simulink model "IO324_src"  (R2022b)
settings: Solver=FixedStepDiscrete  StartTime=0.0  StopTime=10.0  RelTol=1e-3
libraries: SG_library x1, hdlsllib x1
settings Model: DataTypeOverride=Off  Creator=mavolery  LastModifiedBy=mavolery
settings OptimizationCC: BlockReduction=off  ConditionallyExecuteInputs=off  DefaultParameterBehavior=Inlined  InheritOutputTypeSmallerThanSingle=on
settings DebuggingCC: AlgebraicLoopMsg=error  InheritedTsInSrcMsg=none  SingleTaskRateTransMsg=error
settings HardwareCC: ProdBitPerPointer=32  ProdBitPerSizeT=32  ProdBitPerPtrDiffT=32  ProdLargestAtomicFloat=None  ProdIntDivRoundTo=Undefined  ProdEndianess=Unspecified  ProdWordSize=32  ProdHWDeviceType=ASIC/FPGA->ASIC/FPGA  TargetBitPerPointer=64  TargetBitPerSizeT=64  TargetBitPerPtrDiffT=64  TargetLongLongMode=on  TargetIntDivRoundTo=Zero  TargetEndianess=LittleEndian  TargetWordSize=64  TargetHWDeviceType=Custom Processor->MATLAB Host Computer  ProdEqTarget=off

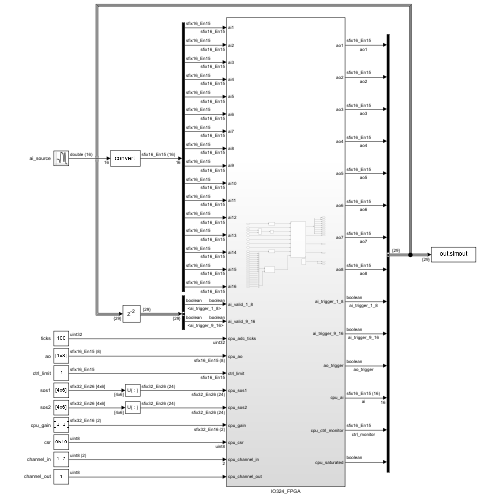
[thumbnail: Simulink's stored preview of the top-level diagram]
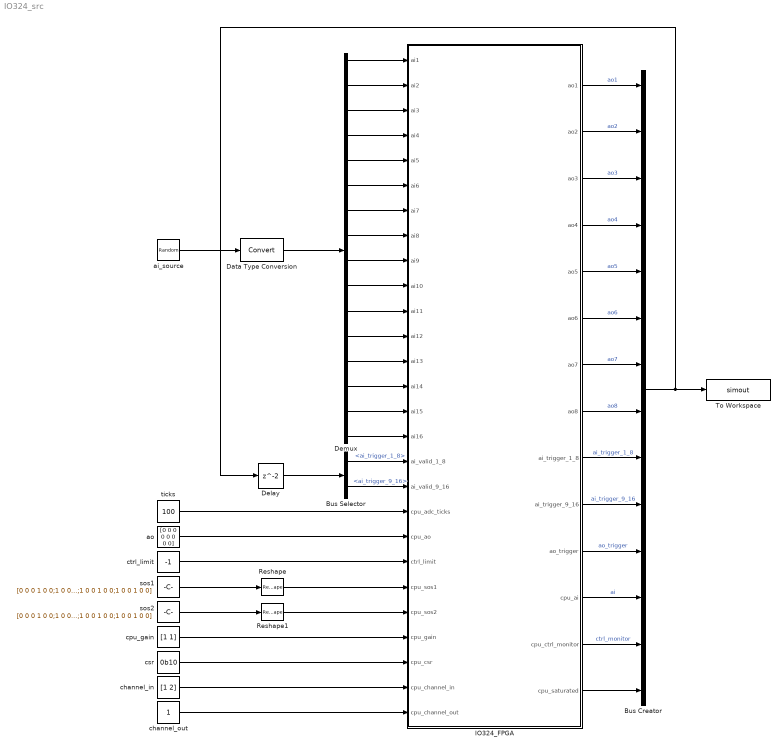
== system IO324_src ==
  Bus Creator : BusCreator  Inputs=14
  Bus Selector : BusSelector  OutputSignals=ai_trigger_1_8,ai_trigger_9_16
  Data Type Conversion : DataTypeConversion  SaturateOnIntegerOverflow=off  RndMeth=Floor
  Delay : Delay
  Demux : Demux  Outputs=16
  IO324_FPGA : Subsystem
  Reshape : Reshape
  Reshape1 : Reshape
  To Workspace : ToWorkspace  VariableName=simout  SaveFormat=Timeseries  SampleTime=-1
  ai_source : RandomNumber  Variance=1e-3  Seed=0:15
  ao : Constant  Value=[0 0 0 0 0 0 0 0]  OutDataTypeStr=Inherit: Inherit via back propagation  SampleTime=-1
  channel_in : Constant  Value=[1 2]  OutDataTypeStr=Inherit: Inherit via back propagation  SampleTime=-1
  channel_out : Constant  OutDataTypeStr=Inherit: Inherit via back propagation  SampleTime=-1
  cpu_gain : Constant  Value=[1 1]  OutDataTypeStr=Inherit: Inherit via back propagation  SampleTime=-1
  csr : Constant  Value=0b10  OutDataTypeStr=Inherit: Inherit via back propagation  SampleTime=-1
  ctrl_limit : Constant  Value=-1  OutDataTypeStr=Inherit: Inherit via back propagation  SampleTime=-1
  sos1 : Constant  Value=[0 0 0 1 0 0;1 0 0 1 0 0;1 0 0 1 0 0;1 0 0 1 0 0]  OutDataTypeStr=Inherit: Inherit via back propagation  SampleTime=-1
  sos2 : Constant  Value=[0 0 0 1 0 0;1 0 0 1 0 0;1 0 0 1 0 0;1 0 0 1 0 0]  OutDataTypeStr=Inherit: Inherit via back propagation  SampleTime=-1
  ticks : Constant  Value=100  OutDataTypeStr=Inherit: Inherit via back propagation  SampleTime=-1
  wires:
  Bus Creator/1 -> To Workspace/1, Delay/1
  IO324_FPGA/12(cpu_ai) -> Bus Creator/12  "ai"
  Reshape/1 -> IO324_FPGA/22(cpu_sos1)
  IO324_FPGA/4(ao4) -> Bus Creator/4  "ao4"
  IO324_FPGA/8(ao8) -> Bus Creator/8  "ao8"
  IO324_FPGA/1(ao1) -> Bus Creator/1  "ao1"
  ctrl_limit/1 -> IO324_FPGA/21(ctrl_limit)
  IO324_FPGA/3(ao3) -> Bus Creator/3  "ao3"
  IO324_FPGA/11(ao_trigger) -> Bus Creator/11  "ao_trigger"
  IO324_FPGA/2(ao2) -> Bus Creator/2  "ao2"
  IO324_FPGA/7(ao7) -> Bus Creator/7  "ao7"
  IO324_FPGA/10(ai_trigger_9_16) -> Bus Creator/10  "ai_trigger_9_16"
  IO324_FPGA/9(ai_trigger_1_8) -> Bus Creator/9  "ai_trigger_1_8"
  IO324_FPGA/13(cpu_ctrl_monitor) -> Bus Creator/13  "ctrl_monitor"
  ticks/1 -> IO324_FPGA/19(cpu_adc_ticks)
  IO324_FPGA/6(ao6) -> Bus Creator/6  "ao6"
  sos2/1 -> Reshape1/1
  csr/1 -> IO324_FPGA/25(cpu_csr)
  cpu_gain/1 -> IO324_FPGA/24(cpu_gain)
  sos1/1 -> Reshape/1
  Reshape1/1 -> IO324_FPGA/23(cpu_sos2)
  IO324_FPGA/5(ao5) -> Bus Creator/5  "ao5"
  ai_source/1 -> Data Type Conversion/1
  ao/1 -> IO324_FPGA/20(cpu_ao)
  Demux/1 -> IO324_FPGA/1(ai1)
  Demux/2 -> IO324_FPGA/2(ai2)
  Demux/3 -> IO324_FPGA/3(ai3)
  Demux/4 -> IO324_FPGA/4(ai4)
  Demux/5 -> IO324_FPGA/5(ai5)
  Demux/6 -> IO324_FPGA/6(ai6)
  Demux/7 -> IO324_FPGA/7(ai7)
  Demux/8 -> IO324_FPGA/8(ai8)
  Demux/9 -> IO324_FPGA/9(ai9)
  Demux/10 -> IO324_FPGA/10(ai10)
  Demux/11 -> IO324_FPGA/11(ai11)
  Demux/12 -> IO324_FPGA/12(ai12)
  Demux/13 -> IO324_FPGA/13(ai13)
  Demux/14 -> IO324_FPGA/14(ai14)
  Demux/15 -> IO324_FPGA/15(ai15)
  Demux/16 -> IO324_FPGA/16(ai16)
  Data Type Conversion/1 -> Demux/1
  Bus Selector/2 -> IO324_FPGA/18(ai_valid_9_16)  "<ai_trigger_9_16>"
  Bus Selector/1 -> IO324_FPGA/17(ai_valid_1_8)  "<ai_trigger_1_8>"
  Delay/1 -> Bus Selector/1
  channel_in/1 -> IO324_FPGA/26(cpu_channel_in)
  channel_out/1 -> IO324_FPGA/27(cpu_channel_out)
  IO324_FPGA/14(cpu_saturated) -> Bus Creator/14

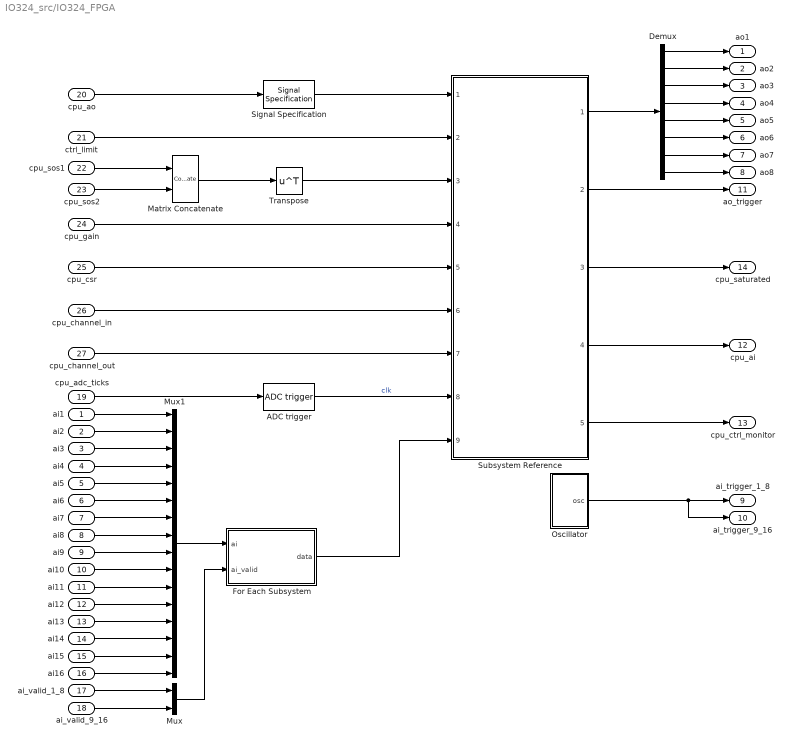
== system IO324_src/IO324_FPGA ==
  ai1 : Inport  OutDataTypeStr=fixdt(1,16,15)
  ai2 : Inport  Port=2  OutDataTypeStr=fixdt(1,16,15)
  ai3 : Inport  Port=3  OutDataTypeStr=fixdt(1,16,15)
  ai4 : Inport  Port=4  OutDataTypeStr=fixdt(1,16,15)
  ai5 : Inport  Port=5  OutDataTypeStr=fixdt(1,16,15)
  ai6 : Inport  Port=6  OutDataTypeStr=fixdt(1,16,15)
  ai7 : Inport  Port=7  OutDataTypeStr=fixdt(1,16,15)
  ai8 : Inport  Port=8  OutDataTypeStr=fixdt(1,16,15)
  ai9 : Inport  Port=9  OutDataTypeStr=fixdt(1,16,15)
  ai10 : Inport  Port=10  OutDataTypeStr=fixdt(1,16,15)
  ai11 : Inport  Port=11  OutDataTypeStr=fixdt(1,16,15)
  ai12 : Inport  Port=12  OutDataTypeStr=fixdt(1,16,15)
  ai13 : Inport  Port=13  OutDataTypeStr=fixdt(1,16,15)
  ai14 : Inport  Port=14  OutDataTypeStr=fixdt(1,16,15)
  ai15 : Inport  Port=15  OutDataTypeStr=fixdt(1,16,15)
  ai16 : Inport  Port=16  OutDataTypeStr=fixdt(1,16,15)
  ai_valid_1_8 : Inport  Port=17  OutDataTypeStr=boolean
  ai_valid_9_16 : Inport  Port=18  OutDataTypeStr=boolean
  cpu_adc_ticks : Inport  Port=19  OutDataTypeStr=uint32
  cpu_ao : Inport  Port=20  OutDataTypeStr=fixdt(1,16,15)
  ctrl_limit : Inport  Port=21  OutDataTypeStr=fixdt(1,16,15)
  cpu_sos1 : Inport  Port=22  OutDataTypeStr=fixdt(1,32,26)
  cpu_sos2 : Inport  Port=23  OutDataTypeStr=fixdt(1,32,26)
  cpu_gain : Inport  Port=24  OutDataTypeStr=fixdt(1,32,16)
  cpu_csr : Inport  Port=25  OutDataTypeStr=uint8
  cpu_channel_in : Inport  Port=26
  cpu_channel_out : Inport  Port=27
  ADC trigger : SG_library/Source elements/ADC trigger
      settings: SourceProductName=Custom Speedgoat implementations
  Demux : Demux  Outputs=8
  For Each Subsystem : Subsystem
  Matrix Concatenate : Concatenate  Mode=Multidimensional array  ConcatenateDimension=2
  Mux : Mux  Inputs=2
  Mux1 : Mux  Inputs=16
  Oscillator : Subsystem
  Signal Specification : SignalSpecification  SampleTime=10e-9
  Subsystem Reference : Subsystem  ReferencedSubsystem=control_filter
  Transpose : Math  Operator=transpose
  ao1 : Outport  VectorParamsAs1DForOutWhenUnconnected=off
  ao2 : Outport  Port=2  VectorParamsAs1DForOutWhenUnconnected=off
  ao3 : Outport  Port=3  VectorParamsAs1DForOutWhenUnconnected=off
  ao4 : Outport  Port=4  VectorParamsAs1DForOutWhenUnconnected=off
  ao5 : Outport  Port=5  VectorParamsAs1DForOutWhenUnconnected=off
  ao6 : Outport  Port=6  VectorParamsAs1DForOutWhenUnconnected=off
  ao7 : Outport  Port=7  VectorParamsAs1DForOutWhenUnconnected=off
  ao8 : Outport  Port=8  VectorParamsAs1DForOutWhenUnconnected=off
  ai_trigger_1_8 : Outport  Port=9  VectorParamsAs1DForOutWhenUnconnected=off
  ai_trigger_9_16 : Outport  Port=10  VectorParamsAs1DForOutWhenUnconnected=off
  ao_trigger : Outport  Port=11  VectorParamsAs1DForOutWhenUnconnected=off
  cpu_ai : Outport  Port=12  VectorParamsAs1DForOutWhenUnconnected=off
  cpu_ctrl_monitor : Outport  Port=13  VectorParamsAs1DForOutWhenUnconnected=off
  cpu_saturated : Outport  Port=14
  wires:
  ai_valid_1_8/1 -> Mux/1
  ai_valid_9_16/1 -> Mux/2
  ai1/1 -> Mux1/1
  ai2/1 -> Mux1/2
  ai3/1 -> Mux1/3
  ai4/1 -> Mux1/4
  ai5/1 -> Mux1/5
  ai6/1 -> Mux1/6
  ai7/1 -> Mux1/7
  ai8/1 -> Mux1/8
  ai9/1 -> Mux1/9
  ai10/1 -> Mux1/10
  ai11/1 -> Mux1/11
  ai12/1 -> Mux1/12
  ai13/1 -> Mux1/13
  ai14/1 -> Mux1/14
  ai15/1 -> Mux1/15
  ai16/1 -> Mux1/16
  Mux1/1 -> For Each Subsystem/1(ai)
  Mux/1 -> For Each Subsystem/2(ai_valid)
  cpu_adc_ticks/1 -> ADC trigger/1
  Demux/1 -> ao1/1
  Demux/2 -> ao2/1
  Demux/3 -> ao3/1
  Demux/4 -> ao4/1
  Demux/5 -> ao5/1
  Demux/6 -> ao6/1
  Demux/7 -> ao7/1
  Demux/8 -> ao8/1
  cpu_ao/1 -> Signal Specification/1
  Subsystem Reference/2 -> ao_trigger/1
  Subsystem Reference/1 -> Demux/1
  Oscillator/1(osc) -> ai_trigger_9_16/1, ai_trigger_1_8/1
  Matrix Concatenate/1 -> Transpose/1
  cpu_sos1/1 -> Matrix Concatenate/1
  cpu_sos2/1 -> Matrix Concatenate/2
  Subsystem Reference/4 -> cpu_ai/1
  Signal Specification/1 -> Subsystem Reference/1
  ctrl_limit/1 -> Subsystem Reference/2
  ADC trigger/1 -> Subsystem Reference/8  "clk"
  Transpose/1 -> Subsystem Reference/3
  cpu_gain/1 -> Subsystem Reference/4
  cpu_csr/1 -> Subsystem Reference/5
  cpu_channel_in/1 -> Subsystem Reference/6
  cpu_channel_out/1 -> Subsystem Reference/7
  For Each Subsystem/1(data) -> Subsystem Reference/9
  Subsystem Reference/3 -> cpu_saturated/1
  Subsystem Reference/5 -> cpu_ctrl_monitor/1

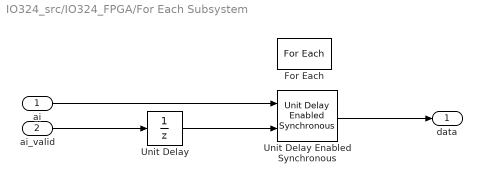
== system IO324_src/IO324_FPGA/For Each Subsystem ==
  ai : Inport  Partition=on  PartitionDimension=1  PartitionWidth=8  PartitionOffset=0
  ai_valid : Inport  Port=2  Partition=on  PartitionDimension=1  PartitionWidth=1  PartitionOffset=0
  For Each : ForEach  DisableCoverage=on
  Unit Delay : UnitDelay  SampleTime=-1  HasFrameUpgradeWarning=on
  Unit Delay Enabled Synchronous : hdlsllib/Discrete/Unit Delay Enabled Synchronous  InitialCondition=0.0  SampleTime=-1
  data : Outport  ConcatenationDimension=1
  wires:
  ai/1 -> Unit Delay Enabled Synchronous/1
  Unit Delay Enabled Synchronous/1 -> data/1
  ai_valid/1 -> Unit Delay/1
  Unit Delay/1 -> Unit Delay Enabled Synchronous/2

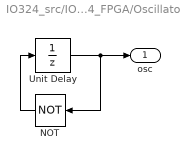
== system IO324_src/IO324_FPGA/Oscillator ==
  NOT : Logic  Operator=NOT  IconShape=distinctive  AllPortsSameDT=off  OutDataTypeStr=boolean
  Unit Delay : UnitDelay  InitialCondition=false  SampleTime=-1  HasFrameUpgradeWarning=on
  osc : Outport
  wires:
  Unit Delay/1 -> NOT/1, osc/1
  NOT/1 -> Unit Delay/1
